simulink model "task2_lab11"  (R2021a)
settings: Solver=VariableStepAuto  StartTime=0.0  StopTime=10.0  RelTol=1e-3
settings Model: Creator=reemb  LastModifiedBy=reemb

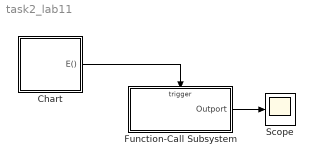
== system task2_lab11 ==
  Chart : Stateflow chart  TreatAsAtomicUnit=on
  Function-Call Subsystem : Subsystem  TreatAsAtomicUnit=on
  Scope : Scope
  wires:
  Chart/1(E()) -> Function-Call Subsystem/Trigger
  Function-Call Subsystem/1(Outport) -> Scope/1

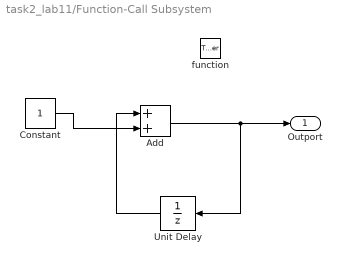
== system task2_lab11/Function-Call Subsystem ==
  function : TriggerPort  TriggerType=function-call  VariantControl=(inherit)
  Add : Sum
  Constant : Constant
  Unit Delay : UnitDelay  SampleTime=-1  HasFrameUpgradeWarning=on
  Outport : Outport
  wires:
  Unit Delay/1 -> Add/1
  Add/1 -> Unit Delay/1, Outport/1
  Constant/1 -> Add/2

== stateflow chart task2_lab11/Chart ==
  state A
    during: E;
  state B
  A -> B : after(1, sec)
  (default) -> A
  B -> A : after(1, sec)
  events: E output FUNCTION_CALL_EVENT
